simulink model "disc_flight_from_ic"  (R2021b)
settings: Solver=ode1be  StartTime=0.0  StopTime=5  FixedStep=0.01  MaxStep=0.01  MinStep=0.01  RelTol=1e-3
values from neighbouring files (symbols this model uses):
  amb = evalin( 'base', 'amb')    [flatball_6dof_eqom.m]
  disc = evalin( 'base', 'disc')    [flatball_6dof_eqom.m]    (also in flatball_6dof_init.m = struct; flatball_init_disc_params.m = struct)
libraries: simulink x1
settings Model: Creator=schae  LastModifiedBy=schae
settings SolverCC: InitialStep=0.01
settings DataIOCC: ReturnWorkspaceOutputsName=simout

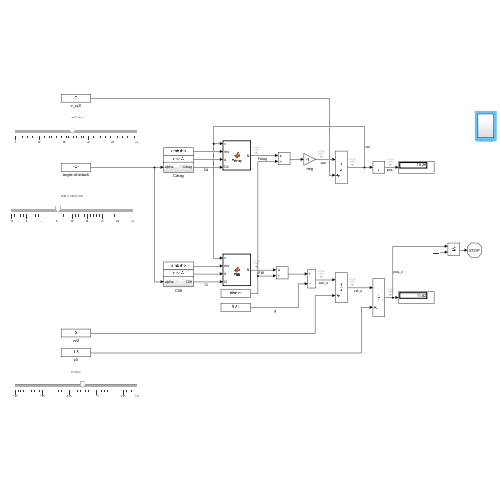
[thumbnail: Simulink's stored preview of the top-level diagram]
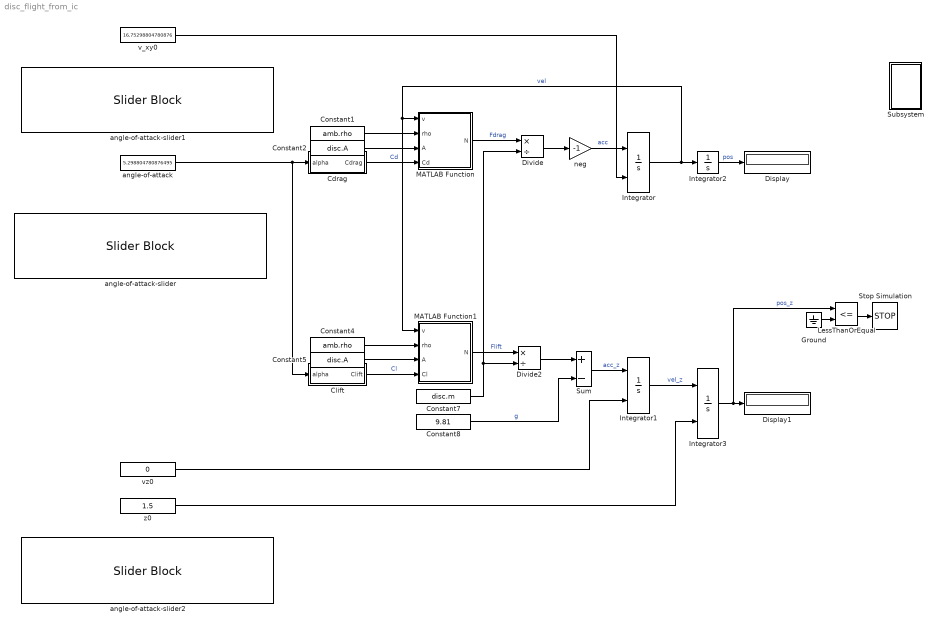
== system disc_flight_from_ic ==
  Cdrag : Subsystem
  Clift : Subsystem
  Constant1 : Constant  Value=amb.rho
  Constant2 : Constant  Value=disc.A
  Constant4 : Constant  Value=amb.rho
  Constant5 : Constant  Value=disc.A
  Constant7 : Constant  Value=disc.m
  Constant8 : Constant  Value=9.81
  Display : Display
  Display1 : Display
  Divide : Product  Inputs=*/
  Divide2 : Product  Inputs=*/
  Ground : Ground
  Integrator : Integrator  InitialConditionSource=external  InitialCondition=15
  Integrator1 : Integrator  InitialConditionSource=external
  Integrator2 : Integrator
  Integrator3 : Integrator  InitialConditionSource=external  InitialCondition=1.5
  LessThanOrEqual : RelationalOperator  Operator=<=  OutDataTypeStr=boolean  RndMeth=Simplest
  MATLAB Function : MATLAB Function  TreatAsAtomicUnit=on
  MATLAB Function1 : MATLAB Function  TreatAsAtomicUnit=on
  Stop Simulation : Stop
  Subsystem : Subsystem
  Sum : Sum  Inputs=+-
  angle-of-attack : Constant  Value=5.298804780876495
  angle-of-attack-slider : SliderBlock  ScaleMin=-10  ScaleMax=30  TickInterval=5
  angle-of-attack-slider1 : SliderBlock  ScaleMin=5  ScaleMax=30  TickInterval=5
  angle-of-attack-slider2 : SliderBlock  ScaleMin=0.25  ScaleMax=2.5  TickInterval=0.5
  neg : Gain  Gain=-1
  v_xy0 : Constant  Value=16.75298804780876
  vz0 : Constant  Value=0
  z0 : Constant  Value=1.5
  wires:
  Constant1/1 -> MATLAB Function/2(rho)
  Constant2/1 -> MATLAB Function/3(A)
  Cdrag/1(Cdrag) -> MATLAB Function/4(Cd)  "Cd"
  Constant4/1 -> MATLAB Function1/2(rho)
  Constant5/1 -> MATLAB Function1/3(A)
  Clift/1(Clift) -> MATLAB Function1/4(Cl)  "Cl"
  Constant7/1 -> Divide/2, Divide2/2
  MATLAB Function/1(N) -> Divide/1  "Fdrag"
  Divide/1 -> neg/1
  Integrator/1 -> MATLAB Function1/1(v), MATLAB Function/1(v), Integrator2/1  "vel"
  neg/1 -> Integrator/1  "acc"
  Sum/1 -> Integrator1/1  "acc_z"
  Integrator1/1 -> Integrator3/1  "vel_z"
  MATLAB Function1/1(N) -> Divide2/1  "Flift"
  Divide2/1 -> Sum/1
  Constant8/1 -> Sum/2  "g"
  Integrator2/1 -> Display/1  "pos"
  Integrator3/1 -> LessThanOrEqual/1, Display1/1  "pos_z"
  LessThanOrEqual/1 -> Stop Simulation/1
  Ground/1 -> LessThanOrEqual/2
  angle-of-attack/1 -> Clift/1(alpha), Cdrag/1(alpha)
  z0/1 -> Integrator3/2
  v_xy0/1 -> Integrator/2
  vz0/1 -> Integrator1/2

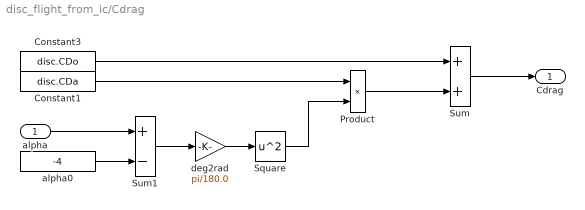
== system disc_flight_from_ic/Cdrag ==
  alpha : Inport
  Constant1 : Constant  Value=disc.CDa
  Constant3 : Constant  Value=disc.CDo
  Product : Product
  Square : Math  Operator=square  SaturateOnIntegerOverflow=on
  Sum : Sum
  Sum1 : Sum  Inputs=+-
  alpha0 : Constant  Value=-4
  deg2rad : Gain  Gain=pi/180.0
  Cdrag : Outport
  wires:
  Constant3/1 -> Sum/1
  alpha/1 -> Sum1/1
  Constant1/1 -> Product/1
  Product/1 -> Sum/2
  alpha0/1 -> Sum1/2
  Sum/1 -> Cdrag/1
  Sum1/1 -> deg2rad/1
  Square/1 -> Product/2
  deg2rad/1 -> Square/1

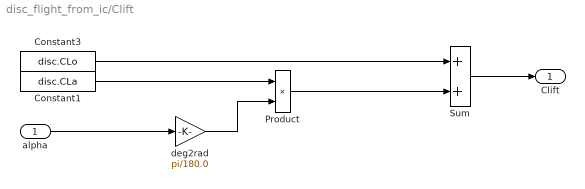
== system disc_flight_from_ic/Clift ==
  alpha : Inport
  Constant1 : Constant  Value=disc.CLa
  Constant3 : Constant  Value=disc.CLo
  Product : Product
  Sum : Sum
  deg2rad : Gain  Gain=pi/180.0
  Clift : Outport
  wires:
  Sum/1 -> Clift/1
  Product/1 -> Sum/2
  Constant1/1 -> Product/1
  Constant3/1 -> Sum/1
  alpha/1 -> deg2rad/1
  deg2rad/1 -> Product/2

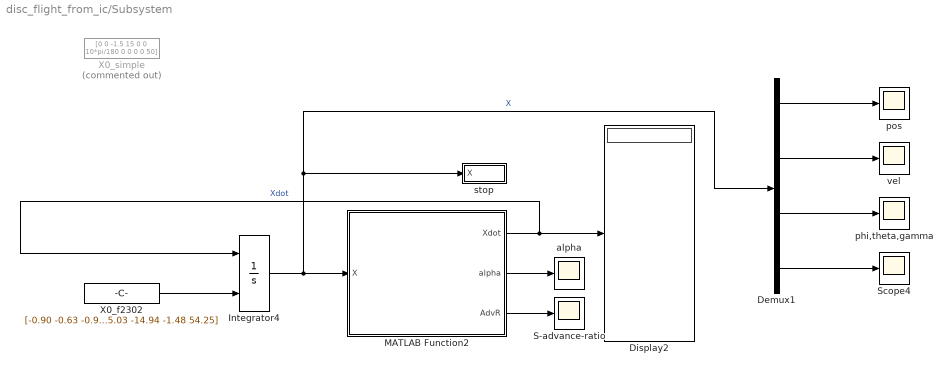
== system disc_flight_from_ic/Subsystem ==
  Demux1 : Demux  Outputs=[3 3 3 3]
  Display2 : Display
  Integrator4 : Integrator  InitialConditionSource=external
  MATLAB Function2 : MATLAB Function  TreatAsAtomicUnit=on
  S-advance-ratio : Scope
  Scope4 : Scope
  X0_f2302 : Constant  Value=[-0.90 -0.63 -0.91 13.42 -0.41 0.001 -0.07 0.21 5.03 -14.94 -1.48 54.25]
  X0_simple : Constant  Commented=on  Value=[0 0 -1.5 15 0 0 10*pi/180 0 0 0 0 50]
  alpha : Scope
  phi,theta,gamma : Scope
  pos : Scope
  stop : Subsystem
  vel : Scope
  wires:
  MATLAB Function2/1(Xdot) -> Integrator4/1, Display2/1  "Xdot"
  X0_f2302/1 -> Integrator4/2
  Demux1/3 -> phi,theta,gamma/1
  Demux1/1 -> pos/1
  Demux1/4 -> Scope4/1
  Demux1/2 -> vel/1
  Integrator4/1 -> Demux1/1, stop/1(X), MATLAB Function2/1(X)  "X"
  MATLAB Function2/2(alpha) -> alpha/1
  MATLAB Function2/3(AdvR) -> S-advance-ratio/1

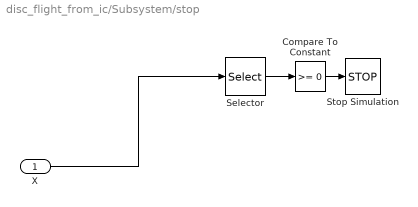
== system disc_flight_from_ic/Subsystem/stop ==
  X : Inport
  Compare To Constant : simulink/Logic and Bit Operations/Compare To Constant  relop=>=  const=0  OutDataTypeStr=boolean
  Selector : Selector  InputPortWidth=12  IndexOptions=Index vector (dialog)  Indices=[3]  OutputSizes=1
  Stop Simulation : Stop
  wires:
  Selector/1 -> Compare To Constant/1
  Compare To Constant/1 -> Stop Simulation/1
  X/1 -> Selector/1

== matlab function disc_flight_from_ic/MATLAB Function1 ==
  data: v input; N output; rho input; A input; Cl input
function N = Flift( v, rho, A, Cl)
% rho = 1.23;
% A = 0.057;
% Cl = 0.3331;

N = 0.5 * rho * v*v * A * Cl;

== matlab function disc_flight_from_ic/MATLAB Function ==
  data: v input; N output; rho input; A input; Cd input
function N = Fdrag( v, rho, A, Cd)
% rho = 1.23;
% A = 0.057;
% Cd = 0.1769;

N = 0.5 * rho * v*v * A * Cd;

== matlab function disc_flight_from_ic/Subsystem/MATLAB Function2 ==
  data: X input; Xdot output; alpha output; AdvR output
function [Xdot, alpha, AdvR]  = flatball_eom( X)
% flatball equations of motion - NED (north-east-down) configuration
%

%% define ambient parameters
amb.g = 9.7935; % m/s^2
amb.rho = 1.23; % Kg/m^3

%% define non-aerodynamic parameters
disc = struct;
disc.m = 0.175; % Kg
disc.A = 0.057; % m^2
disc.d = 2*sqrt(0.057/pi); % 2*sqrt(disc.A/pi); % diameter
disc.Ia = 0.002352; % moment of inertia about the spinning axis
disc.Id = 0.001219; % moment of inertia about the planar axis'

disc.alpha0 = -4 * pi/180.0;

%% THE THREE ESTIMATED COEFFICIENTS
disc.CMq= -1.44E-02;
disc.CRp =-1.25E-02;
disc.CNr = -3.41E-05; % long flight f2302

%% THE seven COEFFICIENTS estimated from three flights
disc.CL0= 0.3331;
disc.CLa= 1.9124;
disc.CD0= 0.1769;
disc.CDa= 0.685;
disc.CM0= -0.0821;
disc.CMa= 0.4338;
disc.CRr= 0.00171; % for nondimensionalization = sqrt(d/g), magnitude of CRr changes

%% internal states
Xdot = zeros(1,12);
x = X(1); y = X(2); z = X(3);
vx = X(4); vy = X(5); vz = X(6);

phi = X(7); theta = X(8); gamma = X(9);
phidot = X(10); thetadot = X(11); gammadot = X(12);

%% helper variables
sin_theta = sin( theta);
cos_theta = cos( theta);
sin_phi = sin( phi);
cos_phi = cos(phi);

% c = T_c_N * N --> transformation matrix T_c_N in N reference frame
T_c_N = [cos_theta sin_theta*sin_phi -sin_theta*cos_phi;
    0 cos_phi sin_phi;
    sin_theta -cos_theta*sin_phi cos_theta*cos_phi];

% [d]=[T_d_N] * [N]
% [e,v] = eig( T_c_N);
% eigM1 = diag(v);
% m1 = norm( eigM1(1));
% m2 = norm( eigM1(2));
% m3 = norm( eigM1(3));
% c1 = T_c_N(1,:);
% c2 = T_c_N(2,:);
c3 = T_c_N(3,:);

%% aerodynamic forces and moments in N reference frame
vel = [vx vy vz];
vmag = norm( vel);
vc3 = dot( vel, c3);
v_N = [ vel - vc3*c3];

Adp = 0.5 * disc.A * amb.rho * vmag*vmag;
uvel = vel / vmag;
uv_N = v_N / norm( v_N);
u_lat = cross( c3, uv_N);

wD_N_inC = [phidot*cos_theta thetadot phidot*sin_theta+gammadot];
wD_N_inN = T_c_N' * wD_N_inC';

w_v_N = dot( wD_N_inN, uv_N);
w_lat = dot( wD_N_inN, u_lat);
w_spin = dot( wD_N_inN, c3);

alpha = atan( vc3 / norm( v_N)); % angle of attack
AdvR = disc.d * w_spin / 2 / vmag; % advance ratio

%% coefficients
Cl = disc.CL0 + disc.CLa * alpha;
dalpha = alpha - disc.alpha0;
Cd = disc.CD0 + disc.CDa * dalpha*dalpha;
Cm = disc.CM0 + disc.CMa * alpha;
Mv_N = Adp * disc.d * (sqrt(disc.d/amb.g)*disc.CRr*w_spin + disc.CRp*w_v_N) * uv_N;

%%
lift = Cl * Adp;
drag = Cd * Adp;
ulift = -cross( uvel, u_lat);
udrag = -uvel;
Faero = lift*ulift + drag*udrag;
Fg_N = [0 0 disc.m*amb.g]';

F = Faero' + Fg_N;

Mlat = Adp * disc.d * (Cm + disc.CMq * w_lat) * u_lat;
Mspin = [0 0 disc.CNr*w_spin];
M = T_c_N * Mv_N' + T_c_N*Mlat' + Mspin';

%%
Xdot(1) = vx; Xdot(2) = vy; Xdot(3) = vz;
Xdot(4) = F(1) / disc.m;
Xdot(5) = F(2) / disc.m;
Xdot(6) = F(3) / disc.m;
Xdot(7) = phidot; Xdot(8) = thetadot; Xdot(9) = gammadot;
Xdot(10) = (M(1) + disc.Id*thetadot*phidot*sin_theta - disc.Ia*thetadot*(phidot*sin_theta+gammadot) + disc.Id*thetadot*phidot*sin_theta)/disc.Id/cos_theta;
phidotdot = Xdot(9);
Xdot(11) = (M(2) + disc.Ia*phidot*cos_theta*(phidot*sin_theta +gammadot) - disc.Id*phidot*phidot*cos_theta*sin_theta)/disc.Id;
Xdot(12) = (M(3) - disc.Ia*(phidotdot*sin_theta + thetadot*phidot*cos_theta))/disc.Ia;
